simulink model "pH_neut_Dynamic"  (R2021b)
settings: Solver=FixedStepAuto  StartTime=0.0  StopTime=2000  FixedStep=0.05  RelTol=1e-3
settings Model: Creator=ismt  LastModifiedBy=ismt

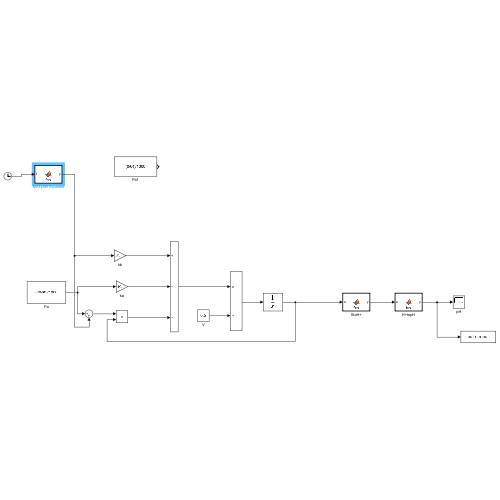
[thumbnail: Simulink's stored preview of the top-level diagram]
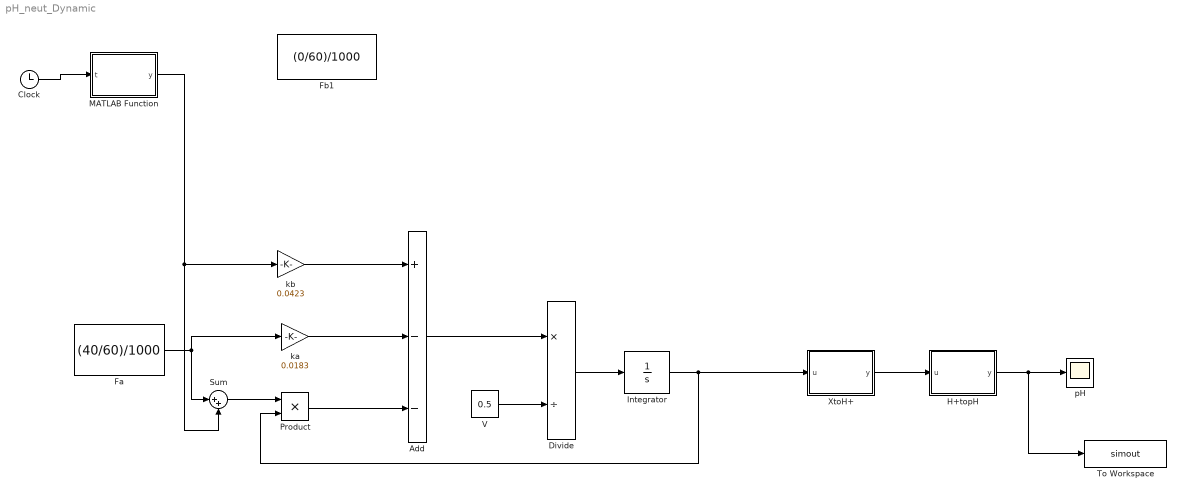
== system pH_neut_Dynamic ==
  Add : Sum  Inputs=+--
  Clock : Clock
  Divide : Product  Inputs=*/
  Fa : Constant  Value=(40/60)/1000
  Fb1 : Constant  Value=(0/60)/1000
  H+topH : MATLAB Function  TreatAsAtomicUnit=on
  Integrator : Integrator
  MATLAB Function : MATLAB Function  TreatAsAtomicUnit=on
  Product : Product
  Sum : Sum  Inputs=|++
  To Workspace : ToWorkspace  VariableName=simout  SaveFormat=Timeseries  SampleTime=-1
  V : Constant  Value=0.5
  XtoH+ : MATLAB Function  TreatAsAtomicUnit=on
  ka : Gain  Gain=0.0183
  kb : Gain  Gain=0.0423
  pH : Scope
  wires:
  MATLAB Function/1(y) -> Sum/2, kb/1
  kb/1 -> Add/1
  Fa/1 -> ka/1, Sum/1
  ka/1 -> Add/2
  Sum/1 -> Product/1
  Integrator/1 -> XtoH+/1(u), Product/2
  Product/1 -> Add/3
  V/1 -> Divide/2
  Add/1 -> Divide/1
  Divide/1 -> Integrator/1
  XtoH+/1(y) -> H+topH/1(u)
  H+topH/1(y) -> To Workspace/1, pH/1
  Clock/1 -> MATLAB Function/1(t)

== matlab function pH_neut_Dynamic/XtoH+ ==
  data: u input; y output
function y = fcn(u)

y = sqrt(((u^2)/4) + 10^(-14))-(u/2);
end

== matlab function pH_neut_Dynamic/MATLAB Function ==
  data: t input; y output
function y = fcn(t)

if t >= 1000
    y = (75/60) / 1000;
else
     y = (10/60) / 1000;
end

== matlab function pH_neut_Dynamic/H+topH ==
  data: u input; y output
function y = fcn(u)

y = -log10(u);
end
